simulink model "RM3_Hydraulic_PTO"  (R2019b)
settings: Solver=ode14x  StartTime=0  StopTime=200  FixedStep=0.0025  MaxStep=0.0025  RelTol=1e-3  EnableMultiTasking=on
undefined symbols (not defined in the file or in its folder): body, DiscIntNeverNeededParam, pto
libraries: fl_lib x1519, nesl_utility x807, sh_lib x675, WECSim_Lib x5
(part 16 of 56)

== system RM3_Hydraulic_PTO/PTO-Sim - Crankshaft DA 4 Cylinders Try 4 WORKS - PR valve no ACCUM - No piston control/Cylinder 2 ==
  Crank Radius : Inport
  Spool Radius : Inport  Port=2
  Angle Displacement : Inport  Port=3
  Crank Init Angle : Inport  Port=4
  Crank Torque [Nm] : Product
  Crank Torque [Nm] Sensor : Scope
  Cyl1 Force Sensor : Scope
  Cylinder 1 to PTO Force convert : Subsystem
  Hydraulic cylinder and valves : Subsystem
  Ideal Translational Motion Sensor : fl_lib/Mechanical/Mechanical Sensors/Ideal Translational Motion Sensor  offset=0 m
  Mass : fl_lib/Mechanical/Translational Elements/Mass  mass=1 kg  v_specify=off  v_priority=High  v=0 m/s  v_nominal_specify=off  v_nominal_unit=m/s  v_nominal_value=1  f_specify=off  f_priority=None  f=0 N  f_nominal_specify=off  f_nominal_unit=N  f_nominal_value=1
  PTO Force Cyl 1 Sensor : Scope
  Slider-Crank : fl_lib/Mechanical/Mechanisms/Slider-Crank  crank=11/2 in  rod=12 in  inertia=0.01 kg*m^2  k=1e6 N/m  b=0.0001 N/(m/s)  theta_specify=on  theta_priority=High  theta=0 rad  theta_nominal_specify=off  theta_nominal_unit=rad  theta_nominal_value=1  w_specify=off  w_priority=Low  w=0 rad/s  w_nominal_specify=off  w_nominal_unit=rad/s  w_nominal_value=1
      settings: SourceProductName=Simscape  SourceProductBaseCode=SS  InternalSimscapePortConfiguration="{\"Bottom\":[],\"Left\":[{\"id\":\"C\",\"label\":\"C\",\"type\":\"foundation.mechanical.rotational.rotational\"}],\"Right\":[{\"id\":\"S\",\"label\":\"S\",\"type\":\"foundation.mechanical.translational.translational\"}],\"Top\":[]}"
  Theta sensor : Scope
  sin(theta) sensor : Scope
  Angular Vel Source : PMIOPort  Side=Left
  Flow Out : PMIOPort  Port=2  Side=Left
  Flow In : PMIOPort  Port=3  Side=Left
  PTO Force : Outport
  wires:
  Crank Torque [Nm]/1 -> Crank Torque [Nm] Sensor/1
  Hydraulic cylinder and valves/1(Force Out) -> Cylinder 1 to PTO Force convert/5(Cylinder Force), Cyl1 Force Sensor/1
  Crank Radius/1 -> Cylinder 1 to PTO Force convert/1(Crank radius), Crank Torque [Nm]/1
  Cylinder 1 to PTO Force convert/3(PTO Force Cyl) -> PTO Force/1, Crank Torque [Nm]/2, PTO Force Cyl 1 Sensor/1
  Cylinder 1 to PTO Force convert/2(sing(theta)) -> sin(theta) sensor/1
  Spool Radius/1 -> Cylinder 1 to PTO Force convert/4(Spool radius)
  Cylinder 1 to PTO Force convert/1(Theta) -> Theta sensor/1
  Crank Init Angle/1 -> Cylinder 1 to PTO Force convert/2(Crank initial angle)
  Angle Displacement/1 -> Cylinder 1 to PTO Force convert/3(Angle disp)
  connections:
  Hydraulic cylinder and valves/LConn1 -- Ideal Translational Motion Sensor/RConn2
  Mass/LConn1 -- Ideal Translational Motion Sensor/RConn1
  Slider-Crank/RConn1 -- Ideal Translational Motion Sensor/LConn1
  Slider-Crank/LConn1 -- Angular Vel Source/RConn1
  Flow In/RConn1 -- Hydraulic cylinder and valves/LConn3
  Hydraulic cylinder and valves/LConn2 -- Flow Out/RConn1

== system RM3_Hydraulic_PTO/PTO-Sim - Crankshaft DA 4 Cylinders Try 4 WORKS - PR valve no ACCUM - No piston control/Cylinder 3 ==
  Crank Radius : Inport
  Spool Radius : Inport  Port=2
  Angle Displacement : Inport  Port=3
  Crank Init Angle : Inport  Port=4
  Crank Torque [Nm] : Product
  Crank Torque [Nm] Sensor : Scope
  Cyl1 Force Sensor : Scope
  Cylinder 1 to PTO Force convert : Subsystem
  Hydraulic cylinder and valves : Subsystem
  Ideal Translational Motion Sensor : fl_lib/Mechanical/Mechanical Sensors/Ideal Translational Motion Sensor  offset=0 m
  Mass : fl_lib/Mechanical/Translational Elements/Mass  mass=1 kg  v_specify=off  v_priority=High  v=0 m/s  v_nominal_specify=off  v_nominal_unit=m/s  v_nominal_value=1  f_specify=off  f_priority=None  f=0 N  f_nominal_specify=off  f_nominal_unit=N  f_nominal_value=1
  PTO Force Cyl 1 Sensor : Scope
  Slider-Crank : fl_lib/Mechanical/Mechanisms/Slider-Crank  crank=11/2 in  rod=12 in  inertia=0.01 kg*m^2  k=1e6 N/m  b=0.0001 N/(m/s)  theta_specify=on  theta_priority=High  theta=3*pi/2 rad  theta_nominal_specify=off  theta_nominal_unit=rad  theta_nominal_value=1  w_specify=off  w_priority=Low  w=0 rad/s  w_nominal_specify=off  w_nominal_unit=rad/s  w_nominal_value=1
      settings: SourceProductName=Simscape  SourceProductBaseCode=SS  InternalSimscapePortConfiguration="{\"Bottom\":[],\"Left\":[{\"id\":\"C\",\"label\":\"C\",\"type\":\"foundation.mechanical.rotational.rotational\"}],\"Right\":[{\"id\":\"S\",\"label\":\"S\",\"type\":\"foundation.mechanical.translational.translational\"}],\"Top\":[]}"
  Theta sensor : Scope
  sin(theta) sensor : Scope
  Angular Vel Source : PMIOPort  Side=Left
  Flow Out : PMIOPort  Port=2  Side=Left
  Flow In : PMIOPort  Port=3  Side=Left
  PTO Force : Outport
  wires:
  Crank Torque [Nm]/1 -> Crank Torque [Nm] Sensor/1
  Hydraulic cylinder and valves/1(Force Out) -> Cylinder 1 to PTO Force convert/5(Cylinder Force), Cyl1 Force Sensor/1
  Crank Radius/1 -> Cylinder 1 to PTO Force convert/1(Crank radius), Crank Torque [Nm]/1
  Cylinder 1 to PTO Force convert/3(PTO Force Cyl) -> PTO Force/1, Crank Torque [Nm]/2, PTO Force Cyl 1 Sensor/1
  Cylinder 1 to PTO Force convert/2(sing(theta)) -> sin(theta) sensor/1
  Spool Radius/1 -> Cylinder 1 to PTO Force convert/4(Spool radius)
  Cylinder 1 to PTO Force convert/1(Theta) -> Theta sensor/1
  Crank Init Angle/1 -> Cylinder 1 to PTO Force convert/2(Crank initial angle)
  Angle Displacement/1 -> Cylinder 1 to PTO Force convert/3(Angle disp)
  connections:
  Hydraulic cylinder and valves/LConn1 -- Ideal Translational Motion Sensor/RConn2
  Mass/LConn1 -- Ideal Translational Motion Sensor/RConn1
  Slider-Crank/RConn1 -- Ideal Translational Motion Sensor/LConn1
  Slider-Crank/LConn1 -- Angular Vel Source/RConn1
  Flow In/RConn1 -- Hydraulic cylinder and valves/LConn3
  Hydraulic cylinder and valves/LConn2 -- Flow Out/RConn1

== system RM3_Hydraulic_PTO/PTO-Sim - Crankshaft DA 4 Cylinders Try 4 WORKS - PR valve no ACCUM - No piston control/Cylinder 4 ==
  Crank Radius : Inport
  Spool Radius : Inport  Port=2
  Angle Displacement : Inport  Port=3
  Crank Init Angle : Inport  Port=4
  Crank Torque [Nm] : Product
  Crank Torque [Nm] Sensor : Scope
  Cyl1 Force Sensor : Scope
  Cylinder 1 to PTO Force convert : Subsystem
  Hydraulic cylinder and valves : Subsystem
  Ideal Translational Motion Sensor : fl_lib/Mechanical/Mechanical Sensors/Ideal Translational Motion Sensor  offset=0 m
  Mass : fl_lib/Mechanical/Translational Elements/Mass  mass=1 kg  v_specify=off  v_priority=High  v=0 m/s  v_nominal_specify=off  v_nominal_unit=m/s  v_nominal_value=1  f_specify=off  f_priority=None  f=0 N  f_nominal_specify=off  f_nominal_unit=N  f_nominal_value=1
  PTO Force Cyl 1 Sensor : Scope
  Slider-Crank : fl_lib/Mechanical/Mechanisms/Slider-Crank  crank=11/2 in  rod=12 in  inertia=0.01 kg*m^2  k=1e6 N/m  b=0.0001 N/(m/s)  theta_specify=on  theta_priority=High  theta=pi rad  theta_nominal_specify=off  theta_nominal_unit=rad  theta_nominal_value=1  w_specify=off  w_priority=Low  w=0 rad/s  w_nominal_specify=off  w_nominal_unit=rad/s  w_nominal_value=1
      settings: SourceProductName=Simscape  SourceProductBaseCode=SS  InternalSimscapePortConfiguration="{\"Bottom\":[],\"Left\":[{\"id\":\"C\",\"label\":\"C\",\"type\":\"foundation.mechanical.rotational.rotational\"}],\"Right\":[{\"id\":\"S\",\"label\":\"S\",\"type\":\"foundation.mechanical.translational.translational\"}],\"Top\":[]}"
  Theta sensor : Scope
  sin(theta) sensor : Scope
  Angular Vel Source : PMIOPort  Side=Left
  Flow Out : PMIOPort  Port=2  Side=Left
  Flow In : PMIOPort  Port=3  Side=Left
  PTO Force : Outport
  wires:
  Crank Torque [Nm]/1 -> Crank Torque [Nm] Sensor/1
  Hydraulic cylinder and valves/1(Force Out) -> Cylinder 1 to PTO Force convert/5(Cylinder Force), Cyl1 Force Sensor/1
  Crank Radius/1 -> Cylinder 1 to PTO Force convert/1(Crank radius), Crank Torque [Nm]/1
  Cylinder 1 to PTO Force convert/3(PTO Force Cyl) -> PTO Force/1, Crank Torque [Nm]/2, PTO Force Cyl 1 Sensor/1
  Cylinder 1 to PTO Force convert/2(sing(theta)) -> sin(theta) sensor/1
  Spool Radius/1 -> Cylinder 1 to PTO Force convert/4(Spool radius)
  Cylinder 1 to PTO Force convert/1(Theta) -> Theta sensor/1
  Crank Init Angle/1 -> Cylinder 1 to PTO Force convert/2(Crank initial angle)
  Angle Displacement/1 -> Cylinder 1 to PTO Force convert/3(Angle disp)
  connections:
  Hydraulic cylinder and valves/LConn1 -- Ideal Translational Motion Sensor/RConn2
  Mass/LConn1 -- Ideal Translational Motion Sensor/RConn1
  Slider-Crank/RConn1 -- Ideal Translational Motion Sensor/LConn1
  Slider-Crank/LConn1 -- Angular Vel Source/RConn1
  Flow In/RConn1 -- Hydraulic cylinder and valves/LConn3
  Hydraulic cylinder and valves/LConn2 -- Flow Out/RConn1

== system RM3_Hydraulic_PTO/PTO-Sim - Crankshaft DA 4 Cylinders Try 4 WORKS - PR valve no ACCUM - No piston control/RO Membrane ==
  " Flow Rate Feed Sensor" : fl_lib/Hydraulic/Hydraulic Sensors/Hydraulic Flow Rate Sensor
      settings: SourceProductName=Simscape
  Brine : fl_lib/Hydraulic/Hydraulic Elements/Hydraulic Reference
      settings: SourceProductName=Simscape
  Brine1 : fl_lib/Hydraulic/Hydraulic Elements/Hydraulic Reference
      settings: SourceProductName=Simscape
  Flow Rate Brine Sensor : fl_lib/Hydraulic/Hydraulic Sensors/Hydraulic Flow Rate Sensor
      settings: SourceProductName=Simscape
  Flow Rate Permeate Sensor : fl_lib/Hydraulic/Hydraulic Sensors/Hydraulic Flow Rate Sensor
      settings: SourceProductName=Simscape
  Flow Restrictor : fl_lib/Hydraulic/Hydraulic Elements/Linear Hydraulic Resistance  resistance=(0.20) * ( 1/((3.812*10^-12)*(7.4 ) ) ) Pa/(m^3/s)  q_specify=off  q_priority=None  q=0.001 m^3/s  q_nominal_specify=off  q_nominal_unit=m^3/s  q_nominal_value=1  p_specify=off  p_priority=None  p=0 Pa  p_nominal_specify=off  p_nominal_unit=Pa  p_nominal_value=1
      settings: SourceProductName=Simscape  SourceProductBaseCode=SS  InternalSimscapePortConfiguration="{\"Bottom\":[],\"Left\":[{\"id\":\"A\",\"label\":\"A\",\"type\":\"foundation.hydraulic.hydraulic\"}],\"Right\":[{\"id\":\"B\",\"label\":\"B\",\"type\":\"foundation.hydraulic.hydraulic\"}],\"Top\":[]}"
  Osmotic Pressure 1 : sh_lib/Valves/Pressure Control Valves/Pressure Relief Valve  valve_area_spec=1  p_diff_TLU=[30.15e5 : 15e3 : 31.35e5] Pa  area_TLU=[1 : 1 : 9] .* 1e-5 m^2  area_max=10*pi*(0.75/2)^2 in^2  pres_set=30 bar  reg_range=2 bar  C_d=0.7  A_leak=1e-12 m^2  lam_spec=1  B_lam=0.999  Re_cr=12  dynamic=0  tau=0.1 s  area_init=1e-12 m^2
      settings: SourceProductName=Simscape Fluids  SourceProductBaseCode=SH  InternalSimscapePortConfiguration="{\"Bottom\":[],\"Left\":[{\"id\":\"A\",\"label\":\"A\",\"type\":\"foundation.hydraulic.hydraulic\"}],\"Right\":[{\"id\":\"B\",\"label\":\"B\",\"type\":\"foundation.hydraulic.hydraulic\"}],\"Top\":[]}"
  P Brine Exit : Scope
  PS Subtract : fl_lib/Physical Signals/Functions/PS Subtract
      settings: SourceProductName=Simscape
  PS-Simulink Converter7 : nesl_utility/PS-Simulink Converter  PhysicalDomain=network_engine_domain  SubClassName=ps_output  LeftPortType=input  RightPortType=output  PseudoPeriodic=off  Frequencies=[]  Unit=inherit  AffineConversion=off
  Permeate : fl_lib/Hydraulic/Hydraulic Elements/Hydraulic Reference
      settings: SourceProductName=Simscape
  Pressure Drop Brine : fl_lib/Hydraulic/Hydraulic Sensors/Hydraulic Pressure Sensor
      settings: SourceProductName=Simscape
  Pressure Drop Permeate : fl_lib/Hydraulic/Hydraulic Sensors/Hydraulic Pressure Sensor
      settings: SourceProductName=Simscape
  Pressure Perm Before : fl_lib/Hydraulic/Hydraulic Sensors/Hydraulic Pressure Sensor
      settings: SourceProductName=Simscape
  Pressure Sensor Brine1 : fl_lib/Hydraulic/Hydraulic Sensors/Hydraulic Pressure Sensor
      settings: SourceProductName=Simscape
  Pressure Sensor Feed : fl_lib/Hydraulic/Hydraulic Sensors/Hydraulic Pressure Sensor
      settings: SourceProductName=Simscape
  RO Membrane1 : fl_lib/Hydraulic/Hydraulic Elements/Linear Hydraulic Resistance  resistance=1/((3.812*10^-12)*(7.4 ) ) Pa/(m^3/s)  q_specify=off  q_priority=None  q=0.001 m^3/s  q_nominal_specify=off  q_nominal_unit=m^3/s  q_nominal_value=1  p_specify=off  p_priority=None  p=0 Pa  p_nominal_specify=off  p_nominal_unit=Pa  p_nominal_value=1
      settings: SourceProductName=Simscape  SourceProductBaseCode=SS  InternalSimscapePortConfiguration="{\"Bottom\":[],\"Left\":[{\"id\":\"A\",\"label\":\"A\",\"type\":\"foundation.hydraulic.hydraulic\"}],\"Right\":[{\"id\":\"B\",\"label\":\"B\",\"type\":\"foundation.hydraulic.hydraulic\"}],\"Top\":[]}"
  Ref1 : fl_lib/Hydraulic/Hydraulic Elements/Hydraulic Reference
      settings: SourceProductName=Simscape
  Ref2 : fl_lib/Hydraulic/Hydraulic Elements/Hydraulic Reference
      settings: SourceProductName=Simscape
  Pressure Perm before RO : PMIOPort  Side=Right
  Pressure Drop Perm : PMIOPort  Port=2  Side=Right
  Flow rate feed : PMIOPort  Port=3  Side=Right
  Flow rate permeate : PMIOPort  Port=4  Side=Right
  Pressure Feed : PMIOPort  Port=5  Side=Right
  Flow in : PMIOPort  Port=6  Side=Left
  Mass flow rate feed : PMIOPort  Port=7  Side=Right
  Mass Flow rate perm : PMIOPort  Port=8  Side=Right
  Flow rate brine : PMIOPort  Port=9  Side=Right
  Mass flow rate brine : PMIOPort  Port=10  Side=Right
  wires:
  PS-Simulink Converter7/1 -> P Brine Exit/1
  connections:
  RO Membrane1/RConn1 -- Pressure Drop Permeate/RConn1 -- Flow Rate Permeate Sensor/LConn1
  " Flow Rate Feed Sensor"/RConn2 -- Pressure Sensor Brine1/LConn1 -- Pressure Drop Brine/LConn1 -- Flow Restrictor/LConn1 -- Osmotic Pressure 1/LConn1
  Pressure Drop Permeate/LConn1 -- RO Membrane1/LConn1 -- Osmotic Pressure 1/RConn1 -- Pressure Perm Before/LConn1
  Pressure Perm Before/RConn1 -- Ref2/LConn1
  Flow Rate Brine Sensor/LConn1 -- Pressure Drop Brine/RConn1 -- Flow Restrictor/RConn1
  " Flow Rate Feed Sensor"/LConn1 -- Pressure Sensor Feed/LConn1 -- Flow in/RConn1
  Flow Rate Permeate Sensor/RConn2 -- Permeate/LConn1
  Pressure Sensor Brine1/RConn1 -- Brine1/LConn1
  " Flow Rate Feed Sensor"/RConn1 -- Flow rate feed/RConn1
  PS Subtract/RConn1 -- PS-Simulink Converter7/LConn1
  Pressure Sensor Feed/RConn2 -- Pressure Feed/RConn1
  Flow Rate Brine Sensor/RConn2 -- Brine/LConn1
  Pressure Sensor Feed/RConn1 -- Ref1/LConn1
  Flow Rate Permeate Sensor/RConn1 -- Flow rate permeate/RConn1
  Pressure Perm before RO/RConn1 -- Pressure Perm Before/RConn2
  Pressure Drop Brine/RConn2 -- PS Subtract/LConn2
  Pressure Sensor Brine1/RConn2 -- PS Subtract/LConn1
  Pressure Drop Permeate/RConn2 -- Pressure Drop Perm/RConn1
  " Flow Rate Feed Sensor"/RConn3 -- Mass flow rate feed/RConn1
  Flow Rate Permeate Sensor/RConn3 -- Mass Flow rate perm/RConn1
  Flow Rate Brine Sensor/RConn1 -- Flow rate brine/RConn1
  Flow Rate Brine Sensor/RConn3 -- Mass flow rate brine/RConn1

== system RM3_Hydraulic_PTO/PTO-Sim - Crankshaft DA 4 Cylinders Try 5 - Cylinder shutoff control - 1/Cylinder 1 ==
  Crank Radius : Inport
  Spool Radius : Inport  Port=2
  Angle Displacement : Inport  Port=3
  Crank Init Angle : Inport  Port=4
  Crank Torque [Nm] : Product
  Crank Torque [Nm] Sensor : Scope
  Cyl1 Force Sensor : Scope
  Cylinder 1 to PTO Force convert : Subsystem
  Hydraulic cylinder and valves : Subsystem
  Ideal Translational Motion Sensor : fl_lib/Mechanical/Mechanical Sensors/Ideal Translational Motion Sensor  offset=0 m
  Mass : fl_lib/Mechanical/Translational Elements/Mass  mass=1 kg  v_specify=off  v_priority=High  v=0 m/s  v_nominal_specify=off  v_nominal_unit=m/s  v_nominal_value=1  f_specify=off  f_priority=None  f=0 N  f_nominal_specify=off  f_nominal_unit=N  f_nominal_value=1
  PTO Force Cyl 1 Sensor : Scope
  Slider-Crank : fl_lib/Mechanical/Mechanisms/Slider-Crank  crank=11/2 in  rod=12 in  inertia=0.01 kg*m^2  k=1e6 N/m  b=0.0001 N/(m/s)  theta_specify=on  theta_priority=High  theta=pi / 2 rad  theta_nominal_specify=off  theta_nominal_unit=rad  theta_nominal_value=1  w_specify=off  w_priority=Low  w=0 rad/s  w_nominal_specify=off  w_nominal_unit=rad/s  w_nominal_value=1
      settings: SourceProductName=Simscape  SourceProductBaseCode=SS  InternalSimscapePortConfiguration="{\"Bottom\":[],\"Left\":[{\"id\":\"C\",\"label\":\"C\",\"type\":\"foundation.mechanical.rotational.rotational\"}],\"Right\":[{\"id\":\"S\",\"label\":\"S\",\"type\":\"foundation.mechanical.translational.translational\"}],\"Top\":[]}"
  Theta sensor : Scope
  sin(theta) sensor : Scope
  Angular Vel Source : PMIOPort  Side=Left
  Flow Out : PMIOPort  Port=2  Side=Left
  Flow In : PMIOPort  Port=3  Side=Left
  PTO Force : Outport
  wires:
  Crank Torque [Nm]/1 -> Crank Torque [Nm] Sensor/1
  Hydraulic cylinder and valves/1(Force Out) -> Cylinder 1 to PTO Force convert/5(Cylinder Force), Cyl1 Force Sensor/1
  Crank Radius/1 -> Cylinder 1 to PTO Force convert/1(Crank radius), Crank Torque [Nm]/1
  Cylinder 1 to PTO Force convert/3(PTO Force Cyl) -> PTO Force/1, Crank Torque [Nm]/2, PTO Force Cyl 1 Sensor/1
  Cylinder 1 to PTO Force convert/2(sing(theta)) -> sin(theta) sensor/1
  Spool Radius/1 -> Cylinder 1 to PTO Force convert/4(Spool radius)
  Cylinder 1 to PTO Force convert/1(Theta) -> Theta sensor/1
  Crank Init Angle/1 -> Cylinder 1 to PTO Force convert/2(Crank initial angle)
  Angle Displacement/1 -> Cylinder 1 to PTO Force convert/3(Angle disp)
  connections:
  Hydraulic cylinder and valves/LConn1 -- Ideal Translational Motion Sensor/RConn2
  Mass/LConn1 -- Ideal Translational Motion Sensor/RConn1
  Slider-Crank/RConn1 -- Ideal Translational Motion Sensor/LConn1
  Slider-Crank/LConn1 -- Angular Vel Source/RConn1
  Flow In/RConn1 -- Hydraulic cylinder and valves/LConn3
  Hydraulic cylinder and valves/LConn2 -- Flow Out/RConn1

== system RM3_Hydraulic_PTO/PTO-Sim - Crankshaft DA 4 Cylinders Try 5 - Cylinder shutoff control - 1/Cylinder 2 ==
  Crank Radius : Inport
  Spool Radius : Inport  Port=2
  Angle Displacement : Inport  Port=3
  Crank Init Angle : Inport  Port=4
  Crank Torque [Nm] : Product
  Crank Torque [Nm] Sensor : Scope
  Cyl1 Force Sensor : Scope
  Cylinder 1 to PTO Force convert : Subsystem
  Hydraulic cylinder and valves : Subsystem
  Ideal Translational Motion Sensor : fl_lib/Mechanical/Mechanical Sensors/Ideal Translational Motion Sensor  offset=0 m
  Mass : fl_lib/Mechanical/Translational Elements/Mass  mass=1 kg  v_specify=off  v_priority=High  v=0 m/s  v_nominal_specify=off  v_nominal_unit=m/s  v_nominal_value=1  f_specify=off  f_priority=None  f=0 N  f_nominal_specify=off  f_nominal_unit=N  f_nominal_value=1
  PTO Force Cyl 1 Sensor : Scope
  Slider-Crank : fl_lib/Mechanical/Mechanisms/Slider-Crank  crank=11/2 in  rod=12 in  inertia=0.01 kg*m^2  k=1e6 N/m  b=0.0001 N/(m/s)  theta_specify=on  theta_priority=High  theta=0 rad  theta_nominal_specify=off  theta_nominal_unit=rad  theta_nominal_value=1  w_specify=off  w_priority=Low  w=0 rad/s  w_nominal_specify=off  w_nominal_unit=rad/s  w_nominal_value=1
      settings: SourceProductName=Simscape  SourceProductBaseCode=SS  InternalSimscapePortConfiguration="{\"Bottom\":[],\"Left\":[{\"id\":\"C\",\"label\":\"C\",\"type\":\"foundation.mechanical.rotational.rotational\"}],\"Right\":[{\"id\":\"S\",\"label\":\"S\",\"type\":\"foundation.mechanical.translational.translational\"}],\"Top\":[]}"
  Theta sensor : Scope
  sin(theta) sensor : Scope
  Angular Vel Source : PMIOPort  Side=Left
  Flow Out : PMIOPort  Port=2  Side=Left
  Flow In : PMIOPort  Port=3  Side=Left
  PTO Force : Outport
  wires:
  Crank Torque [Nm]/1 -> Crank Torque [Nm] Sensor/1
  Hydraulic cylinder and valves/1(Force Out) -> Cylinder 1 to PTO Force convert/5(Cylinder Force), Cyl1 Force Sensor/1
  Crank Radius/1 -> Cylinder 1 to PTO Force convert/1(Crank radius), Crank Torque [Nm]/1
  Cylinder 1 to PTO Force convert/3(PTO Force Cyl) -> PTO Force/1, Crank Torque [Nm]/2, PTO Force Cyl 1 Sensor/1
  Cylinder 1 to PTO Force convert/2(sing(theta)) -> sin(theta) sensor/1
  Spool Radius/1 -> Cylinder 1 to PTO Force convert/4(Spool radius)
  Cylinder 1 to PTO Force convert/1(Theta) -> Theta sensor/1
  Crank Init Angle/1 -> Cylinder 1 to PTO Force convert/2(Crank initial angle)
  Angle Displacement/1 -> Cylinder 1 to PTO Force convert/3(Angle disp)
  connections:
  Hydraulic cylinder and valves/LConn1 -- Ideal Translational Motion Sensor/RConn2
  Mass/LConn1 -- Ideal Translational Motion Sensor/RConn1
  Slider-Crank/RConn1 -- Ideal Translational Motion Sensor/LConn1
  Slider-Crank/LConn1 -- Angular Vel Source/RConn1
  Flow In/RConn1 -- Hydraulic cylinder and valves/LConn3
  Hydraulic cylinder and valves/LConn2 -- Flow Out/RConn1

== system RM3_Hydraulic_PTO/PTO-Sim - Crankshaft DA 4 Cylinders Try 5 - Cylinder shutoff control - 1/Cylinder 3 ==
  Crank Radius : Inport
  Spool Radius : Inport  Port=2
  Angle Displacement : Inport  Port=3
  Crank Init Angle : Inport  Port=4
  Crank Torque [Nm] : Product
  Crank Torque [Nm] Sensor : Scope
  Cyl1 Force Sensor : Scope
  Cylinder 1 to PTO Force convert : Subsystem
  Hydraulic cylinder and valves : Subsystem
  Ideal Translational Motion Sensor : fl_lib/Mechanical/Mechanical Sensors/Ideal Translational Motion Sensor  offset=0 m
  Mass : fl_lib/Mechanical/Translational Elements/Mass  mass=1 kg  v_specify=off  v_priority=High  v=0 m/s  v_nominal_specify=off  v_nominal_unit=m/s  v_nominal_value=1  f_specify=off  f_priority=None  f=0 N  f_nominal_specify=off  f_nominal_unit=N  f_nominal_value=1
  PTO Force Cyl 1 Sensor : Scope
  Slider-Crank : fl_lib/Mechanical/Mechanisms/Slider-Crank  crank=11/2 in  rod=12 in  inertia=0.01 kg*m^2  k=1e6 N/m  b=0.0001 N/(m/s)  theta_specify=on  theta_priority=High  theta=3*pi/2 rad  theta_nominal_specify=off  theta_nominal_unit=rad  theta_nominal_value=1  w_specify=off  w_priority=Low  w=0 rad/s  w_nominal_specify=off  w_nominal_unit=rad/s  w_nominal_value=1
      settings: SourceProductName=Simscape  SourceProductBaseCode=SS  InternalSimscapePortConfiguration="{\"Bottom\":[],\"Left\":[{\"id\":\"C\",\"label\":\"C\",\"type\":\"foundation.mechanical.rotational.rotational\"}],\"Right\":[{\"id\":\"S\",\"label\":\"S\",\"type\":\"foundation.mechanical.translational.translational\"}],\"Top\":[]}"
  Theta sensor : Scope
  sin(theta) sensor : Scope
  Angular Vel Source : PMIOPort  Side=Left
  Flow Out : PMIOPort  Port=2  Side=Left
  Flow In : PMIOPort  Port=3  Side=Left
  PTO Force : Outport
  wires:
  Crank Torque [Nm]/1 -> Crank Torque [Nm] Sensor/1
  Hydraulic cylinder and valves/1(Force Out) -> Cylinder 1 to PTO Force convert/5(Cylinder Force), Cyl1 Force Sensor/1
  Crank Radius/1 -> Cylinder 1 to PTO Force convert/1(Crank radius), Crank Torque [Nm]/1
  Cylinder 1 to PTO Force convert/3(PTO Force Cyl) -> PTO Force/1, Crank Torque [Nm]/2, PTO Force Cyl 1 Sensor/1
  Cylinder 1 to PTO Force convert/2(sing(theta)) -> sin(theta) sensor/1
  Spool Radius/1 -> Cylinder 1 to PTO Force convert/4(Spool radius)
  Cylinder 1 to PTO Force convert/1(Theta) -> Theta sensor/1
  Crank Init Angle/1 -> Cylinder 1 to PTO Force convert/2(Crank initial angle)
  Angle Displacement/1 -> Cylinder 1 to PTO Force convert/3(Angle disp)
  connections:
  Hydraulic cylinder and valves/LConn1 -- Ideal Translational Motion Sensor/RConn2
  Mass/LConn1 -- Ideal Translational Motion Sensor/RConn1
  Slider-Crank/RConn1 -- Ideal Translational Motion Sensor/LConn1
  Slider-Crank/LConn1 -- Angular Vel Source/RConn1
  Flow In/RConn1 -- Hydraulic cylinder and valves/LConn3
  Hydraulic cylinder and valves/LConn2 -- Flow Out/RConn1

== system RM3_Hydraulic_PTO/PTO-Sim - Crankshaft DA 4 Cylinders Try 5 - Cylinder shutoff control - 1/Cylinder 4 ==
  Crank Radius : Inport
  Spool Radius : Inport  Port=2
  Angle Displacement : Inport  Port=3
  Crank Init Angle : Inport  Port=4
  Crank Torque [Nm] : Product
  Crank Torque [Nm] Sensor : Scope
  Cyl1 Force Sensor : Scope
  Cylinder 1 to PTO Force convert : Subsystem
  Hydraulic cylinder and valves : Subsystem
  Ideal Translational Motion Sensor : fl_lib/Mechanical/Mechanical Sensors/Ideal Translational Motion Sensor  offset=0 m
  Mass : fl_lib/Mechanical/Translational Elements/Mass  mass=1 kg  v_specify=off  v_priority=High  v=0 m/s  v_nominal_specify=off  v_nominal_unit=m/s  v_nominal_value=1  f_specify=off  f_priority=None  f=0 N  f_nominal_specify=off  f_nominal_unit=N  f_nominal_value=1
  PTO Force Cyl 1 Sensor : Scope
  Slider-Crank : fl_lib/Mechanical/Mechanisms/Slider-Crank  crank=11/2 in  rod=12 in  inertia=0.01 kg*m^2  k=1e6 N/m  b=0.0001 N/(m/s)  theta_specify=on  theta_priority=High  theta=pi rad  theta_nominal_specify=off  theta_nominal_unit=rad  theta_nominal_value=1  w_specify=off  w_priority=Low  w=0 rad/s  w_nominal_specify=off  w_nominal_unit=rad/s  w_nominal_value=1
      settings: SourceProductName=Simscape  SourceProductBaseCode=SS  InternalSimscapePortConfiguration="{\"Bottom\":[],\"Left\":[{\"id\":\"C\",\"label\":\"C\",\"type\":\"foundation.mechanical.rotational.rotational\"}],\"Right\":[{\"id\":\"S\",\"label\":\"S\",\"type\":\"foundation.mechanical.translational.translational\"}],\"Top\":[]}"
  Theta sensor : Scope
  sin(theta) sensor : Scope
  Angular Vel Source : PMIOPort  Side=Left
  Flow Out : PMIOPort  Port=2  Side=Left
  Flow In : PMIOPort  Port=3  Side=Left
  PTO Force : Outport
  wires:
  Crank Torque [Nm]/1 -> Crank Torque [Nm] Sensor/1
  Hydraulic cylinder and valves/1(Force Out) -> Cylinder 1 to PTO Force convert/5(Cylinder Force), Cyl1 Force Sensor/1
  Crank Radius/1 -> Cylinder 1 to PTO Force convert/1(Crank radius), Crank Torque [Nm]/1
  Cylinder 1 to PTO Force convert/3(PTO Force Cyl) -> PTO Force/1, Crank Torque [Nm]/2, PTO Force Cyl 1 Sensor/1
  Cylinder 1 to PTO Force convert/2(sing(theta)) -> sin(theta) sensor/1
  Spool Radius/1 -> Cylinder 1 to PTO Force convert/4(Spool radius)
  Cylinder 1 to PTO Force convert/1(Theta) -> Theta sensor/1
  Crank Init Angle/1 -> Cylinder 1 to PTO Force convert/2(Crank initial angle)
  Angle Displacement/1 -> Cylinder 1 to PTO Force convert/3(Angle disp)
  connections:
  Hydraulic cylinder and valves/LConn1 -- Ideal Translational Motion Sensor/RConn2
  Mass/LConn1 -- Ideal Translational Motion Sensor/RConn1
  Slider-Crank/RConn1 -- Ideal Translational Motion Sensor/LConn1
  Slider-Crank/LConn1 -- Angular Vel Source/RConn1
  Flow In/RConn1 -- Hydraulic cylinder and valves/LConn3
  Hydraulic cylinder and valves/LConn2 -- Flow Out/RConn1

== system RM3_Hydraulic_PTO/PTO-Sim - Crankshaft DA 4 Cylinders Try 5 - Cylinder shutoff control - 1/RO Membrane ==
  " Flow Rate Feed Sensor" : fl_lib/Hydraulic/Hydraulic Sensors/Hydraulic Flow Rate Sensor
      settings: SourceProductName=Simscape
  Brine : fl_lib/Hydraulic/Hydraulic Elements/Hydraulic Reference
      settings: SourceProductName=Simscape
  Brine1 : fl_lib/Hydraulic/Hydraulic Elements/Hydraulic Reference
      settings: SourceProductName=Simscape
  Flow Rate Brine Sensor : fl_lib/Hydraulic/Hydraulic Sensors/Hydraulic Flow Rate Sensor
      settings: SourceProductName=Simscape
  Flow Rate Permeate Sensor : fl_lib/Hydraulic/Hydraulic Sensors/Hydraulic Flow Rate Sensor
      settings: SourceProductName=Simscape
  Flow Restrictor : fl_lib/Hydraulic/Hydraulic Elements/Linear Hydraulic Resistance  resistance=(0.30) * ( 1/((3.812*10^-12)*(7.4 ) ) ) Pa/(m^3/s)  q_specify=off  q_priority=None  q=0.001 m^3/s  q_nominal_specify=off  q_nominal_unit=m^3/s  q_nominal_value=1  p_specify=off  p_priority=None  p=0 Pa  p_nominal_specify=off  p_nominal_unit=Pa  p_nominal_value=1
      settings: SourceProductName=Simscape  SourceProductBaseCode=SS  InternalSimscapePortConfiguration="{\"Bottom\":[],\"Left\":[{\"id\":\"A\",\"label\":\"A\",\"type\":\"foundation.hydraulic.hydraulic\"}],\"Right\":[{\"id\":\"B\",\"label\":\"B\",\"type\":\"foundation.hydraulic.hydraulic\"}],\"Top\":[]}"
  Osmotic Pressure 1 : sh_lib/Valves/Pressure Control Valves/Pressure Relief Valve  valve_area_spec=1  p_diff_TLU=[30.15e5 : 15e3 : 31.35e5] Pa  area_TLU=[1 : 1 : 9] .* 1e-5 m^2  area_max=10*pi*(0.75/2)^2 in^2  pres_set=30 bar  reg_range=2 bar  C_d=0.7  A_leak=1e-12 m^2  lam_spec=1  B_lam=0.999  Re_cr=12  dynamic=0  tau=0.1 s  area_init=1e-12 m^2
      settings: SourceProductName=Simscape Fluids  SourceProductBaseCode=SH  InternalSimscapePortConfiguration="{\"Bottom\":[],\"Left\":[{\"id\":\"A\",\"label\":\"A\",\"type\":\"foundation.hydraulic.hydraulic\"}],\"Right\":[{\"id\":\"B\",\"label\":\"B\",\"type\":\"foundation.hydraulic.hydraulic\"}],\"Top\":[]}"
  P Brine Exit : Scope
  PS Subtract : fl_lib/Physical Signals/Functions/PS Subtract
      settings: SourceProductName=Simscape
  PS-Simulink Converter7 : nesl_utility/PS-Simulink Converter  PhysicalDomain=network_engine_domain  SubClassName=ps_output  LeftPortType=input  RightPortType=output  PseudoPeriodic=off  Frequencies=[]  Unit=inherit  AffineConversion=off
  Permeate : fl_lib/Hydraulic/Hydraulic Elements/Hydraulic Reference
      settings: SourceProductName=Simscape
  Pressure Drop Brine : fl_lib/Hydraulic/Hydraulic Sensors/Hydraulic Pressure Sensor
      settings: SourceProductName=Simscape
  Pressure Drop Permeate : fl_lib/Hydraulic/Hydraulic Sensors/Hydraulic Pressure Sensor
      settings: SourceProductName=Simscape
  Pressure Perm Before : fl_lib/Hydraulic/Hydraulic Sensors/Hydraulic Pressure Sensor
      settings: SourceProductName=Simscape
  Pressure Sensor Brine1 : fl_lib/Hydraulic/Hydraulic Sensors/Hydraulic Pressure Sensor
      settings: SourceProductName=Simscape
  Pressure Sensor Feed : fl_lib/Hydraulic/Hydraulic Sensors/Hydraulic Pressure Sensor
      settings: SourceProductName=Simscape
  RO Membrane1 : fl_lib/Hydraulic/Hydraulic Elements/Linear Hydraulic Resistance  resistance=1/((3.812*10^-12)*(7.4 ) ) Pa/(m^3/s)  q_specify=off  q_priority=None  q=0.001 m^3/s  q_nominal_specify=off  q_nominal_unit=m^3/s  q_nominal_value=1  p_specify=off  p_priority=None  p=0 Pa  p_nominal_specify=off  p_nominal_unit=Pa  p_nominal_value=1
      settings: SourceProductName=Simscape  SourceProductBaseCode=SS  InternalSimscapePortConfiguration="{\"Bottom\":[],\"Left\":[{\"id\":\"A\",\"label\":\"A\",\"type\":\"foundation.hydraulic.hydraulic\"}],\"Right\":[{\"id\":\"B\",\"label\":\"B\",\"type\":\"foundation.hydraulic.hydraulic\"}],\"Top\":[]}"
  Ref1 : fl_lib/Hydraulic/Hydraulic Elements/Hydraulic Reference
      settings: SourceProductName=Simscape
  Ref2 : fl_lib/Hydraulic/Hydraulic Elements/Hydraulic Reference
      settings: SourceProductName=Simscape
  Pressure Perm before RO : PMIOPort  Side=Right
  Pressure Drop Perm : PMIOPort  Port=2  Side=Right
  Flow rate feed : PMIOPort  Port=3  Side=Right
  Flow rate permeate : PMIOPort  Port=4  Side=Right
  Pressure Feed : PMIOPort  Port=5  Side=Right
  Flow in : PMIOPort  Port=6  Side=Left
  Mass flow rate feed : PMIOPort  Port=7  Side=Right
  Mass Flow rate perm : PMIOPort  Port=8  Side=Right
  Flow rate brine : PMIOPort  Port=9  Side=Right
  Mass flow rate brine : PMIOPort  Port=10  Side=Right
  wires:
  PS-Simulink Converter7/1 -> P Brine Exit/1
  connections:
  RO Membrane1/RConn1 -- Pressure Drop Permeate/RConn1 -- Flow Rate Permeate Sensor/LConn1
  " Flow Rate Feed Sensor"/RConn2 -- Pressure Sensor Brine1/LConn1 -- Pressure Drop Brine/LConn1 -- Flow Restrictor/LConn1 -- Osmotic Pressure 1/LConn1
  Pressure Drop Permeate/LConn1 -- RO Membrane1/LConn1 -- Osmotic Pressure 1/RConn1 -- Pressure Perm Before/LConn1
  Pressure Perm Before/RConn1 -- Ref2/LConn1
  Flow Rate Brine Sensor/LConn1 -- Pressure Drop Brine/RConn1 -- Flow Restrictor/RConn1
  " Flow Rate Feed Sensor"/LConn1 -- Pressure Sensor Feed/LConn1 -- Flow in/RConn1
  Flow Rate Permeate Sensor/RConn2 -- Permeate/LConn1
  Pressure Sensor Brine1/RConn1 -- Brine1/LConn1
  " Flow Rate Feed Sensor"/RConn1 -- Flow rate feed/RConn1
  PS Subtract/RConn1 -- PS-Simulink Converter7/LConn1
  Pressure Sensor Feed/RConn2 -- Pressure Feed/RConn1
  Flow Rate Brine Sensor/RConn2 -- Brine/LConn1
  Pressure Sensor Feed/RConn1 -- Ref1/LConn1
  Flow Rate Permeate Sensor/RConn1 -- Flow rate permeate/RConn1
  Pressure Perm before RO/RConn1 -- Pressure Perm Before/RConn2
  Pressure Drop Brine/RConn2 -- PS Subtract/LConn2
  Pressure Sensor Brine1/RConn2 -- PS Subtract/LConn1
  Pressure Drop Permeate/RConn2 -- Pressure Drop Perm/RConn1
  " Flow Rate Feed Sensor"/RConn3 -- Mass flow rate feed/RConn1
  Flow Rate Permeate Sensor/RConn3 -- Mass Flow rate perm/RConn1
  Flow Rate Brine Sensor/RConn1 -- Flow rate brine/RConn1
  Flow Rate Brine Sensor/RConn3 -- Mass flow rate brine/RConn1

== system RM3_Hydraulic_PTO/PTO-Sim - Crankshaft DA 4 Cylinders Try 5 - Cylinder shutoff control - 1/Water Quality Block ==
  A_w/Bs : fl_lib/Physical Signals/Functions/PS Gain  gain=3.812*10^(-12)/(6.986*10^(-8))
  C_m : fl_lib/Physical Signals/Sources/PS Constant  constant=35000
  Constant : Constant  Value=0
  Cp : Scope  NumInputPorts=2
  Divide : Product
  If : If
  If Action Perm Flow  > 0 : Subsystem  TreatAsAtomicUnit=on
  If Action Subsystem1 : Subsystem  TreatAsAtomicUnit=on
  P Permeate Exit : Scope
  PS Add : fl_lib/Physical Signals/Functions/PS Add
  PS Constant : fl_lib/Physical Signals/Sources/PS Constant  constant=1 Pa
  PS Divide : fl_lib/Physical Signals/Functions/PS Divide
      settings: SourceProductName=Simscape  SourceProductBaseCode=SS
  PS Subtract1 : fl_lib/Physical Signals/Functions/PS Subtract
      settings: SourceProductName=Simscape
  PS-Simulink Converter{5..6,8..11} (6 alike) : nesl_utility/PS-Simulink Converter  PhysicalDomain=network_engine_domain  SubClassName=ps_output  LeftPortType=input  RightPortType=output  PseudoPeriodic=off  Frequencies=[]  Unit=inherit  AffineConversion=off
  Permeate Cp*Flow : Scope
  Recov Ratio : fl_lib/Physical Signals/Functions/PS Divide
      settings: SourceProductName=Simscape  SourceProductBaseCode=SS
  Recov Ratio % : Scope
  Pressure Perm Before : PMIOPort  Side=Left
  Pressure Dop Permeate : PMIOPort  Port=2  Side=Left
  Flow rate feed sensor : PMIOPort  Port=3  Side=Left
  Flow rate permeate : PMIOPort  Port=4  Side=Left
  wires:
  If Action Perm Flow  > 0/1(Out1) -> Cp/2
  Divide/1 -> Permeate Cp*Flow/1
  If/1 -> If Action Perm Flow  > 0/Action
  If Action Subsystem1/1(Out1) -> Cp/1
  If/2 -> If Action Subsystem1/Action
  PS-Simulink Converter10/1 -> Divide/1
  PS-Simulink Converter9/1 -> If/1
  PS-Simulink Converter8/1 -> P Permeate Exit/1
  PS-Simulink Converter6/1 -> Recov Ratio %/1
  PS-Simulink Converter11/1 -> Divide/2
  Constant/1 -> If Action Subsystem1/1(In1)
  PS-Simulink Converter5/1 -> If Action Perm Flow  > 0/1(In1)
  connections:
  A_w/Bs/LConn1 -- PS-Simulink Converter9/LConn1 -- PS Subtract1/LConn1 -- Pressure Perm Before/RConn1
  PS Divide/RConn1 -- PS-Simulink Converter5/LConn1 -- PS-Simulink Converter10/LConn1
  Recov Ratio/RConn1 -- PS-Simulink Converter6/LConn1
  PS Constant/RConn1 -- PS Add/LConn2
  Recov Ratio/LConn1 -- PS-Simulink Converter11/LConn1 -- Flow rate permeate/RConn1
  PS Subtract1/RConn1 -- PS-Simulink Converter8/LConn1
  PS Add/LConn1 -- A_w/Bs/RConn1
  C_m/RConn1 -- PS Divide/LConn1
  PS Divide/LConn2 -- PS Add/RConn1
  Flow rate feed sensor/RConn1 -- Recov Ratio/LConn2
  Pressure Dop Permeate/RConn1 -- PS Subtract1/LConn2

== system RM3_Hydraulic_PTO/PTO-Sim - Crankshaft DA Cylinder - doesn't work/Water Quality Block ==
  A_w/Bs : fl_lib/Physical Signals/Functions/PS Gain  gain=3.812*10^(-12)/(6.986*10^(-8))
  C_m : fl_lib/Physical Signals/Sources/PS Constant  constant=35000
  Constant : Constant  Value=0
  Cp : Scope  NumInputPorts=2
  Divide : Product
  If : If
  If Action Perm Flow  > 0 : Subsystem  TreatAsAtomicUnit=on
  If Action Subsystem1 : Subsystem  TreatAsAtomicUnit=on
  P Permeate Exit : Scope
  PS Add : fl_lib/Physical Signals/Functions/PS Add
  PS Constant : fl_lib/Physical Signals/Sources/PS Constant  constant=1 Pa
  PS Divide : fl_lib/Physical Signals/Functions/PS Divide
      settings: SourceProductName=Simscape  SourceProductBaseCode=SS
  PS Subtract1 : fl_lib/Physical Signals/Functions/PS Subtract
      settings: SourceProductName=Simscape
  PS-Simulink Converter{5..6,8..11} (6 alike) : nesl_utility/PS-Simulink Converter  PhysicalDomain=network_engine_domain  SubClassName=ps_output  LeftPortType=input  RightPortType=output  PseudoPeriodic=off  Frequencies=[]  Unit=inherit  AffineConversion=off
  Permeate Cp*Flow : Scope
  Recov Ratio : fl_lib/Physical Signals/Functions/PS Divide
      settings: SourceProductName=Simscape  SourceProductBaseCode=SS
  Recov Ratio % : Scope
  Pressure Perm Before : PMIOPort  Side=Left
  Pressure Dop Permeate : PMIOPort  Port=2  Side=Left
  Flow rate feed sensor : PMIOPort  Port=3  Side=Left
  Flow rate permeate : PMIOPort  Port=4  Side=Left
  wires:
  If Action Perm Flow  > 0/1(Out1) -> Cp/2
  Divide/1 -> Permeate Cp*Flow/1
  If/1 -> If Action Perm Flow  > 0/Action
  If Action Subsystem1/1(Out1) -> Cp/1
  If/2 -> If Action Subsystem1/Action
  PS-Simulink Converter10/1 -> Divide/1
  PS-Simulink Converter9/1 -> If/1
  PS-Simulink Converter8/1 -> P Permeate Exit/1
  PS-Simulink Converter6/1 -> Recov Ratio %/1
  PS-Simulink Converter11/1 -> Divide/2
  Constant/1 -> If Action Subsystem1/1(In1)
  PS-Simulink Converter5/1 -> If Action Perm Flow  > 0/1(In1)
  connections:
  A_w/Bs/LConn1 -- PS-Simulink Converter9/LConn1 -- Pressure Perm Before/RConn1 -- PS Subtract1/LConn1
  PS Divide/RConn1 -- PS-Simulink Converter5/LConn1 -- PS-Simulink Converter10/LConn1
  Recov Ratio/RConn1 -- PS-Simulink Converter6/LConn1
  PS Constant/RConn1 -- PS Add/LConn2
  Recov Ratio/LConn1 -- Flow rate permeate/RConn1 -- PS-Simulink Converter11/LConn1
  PS Subtract1/RConn1 -- PS-Simulink Converter8/LConn1
  PS Add/LConn1 -- A_w/Bs/RConn1
  C_m/RConn1 -- PS Divide/LConn1
  PS Divide/LConn2 -- PS Add/RConn1
  Flow rate feed sensor/RConn1 -- Recov Ratio/LConn2
  Pressure Dop Permeate/RConn1 -- PS Subtract1/LConn2

== system RM3_Hydraulic_PTO/PTO-Sim - Crankshaft DA Cylinder Try 2 - WORKS!1/Hydraulic cylinder and valves ==
  3 Way Directional Valve : sh_lib/Valves/Directional Valves/3-Way Directional Valve  area_spec=sh.valves.directional_valves.enum.area_spec.identical  x_0_P=0 m  x_0_T=0 m  mdl_type_identical=sh.valves.directional_valves.enum.mdl_type.linear  mdl_type_different=sh.valves.directional_valves.enum.mdl_type.linear  opening_max=0.75 in  area_max=pi*(0.75/2)^2 in^2  opening_max_P_A=0.005 m  area_max_P_A=0.5e-4 m^2  opening_max_A_T=0.005 m  area_max_A_T=0.5e-4 m^2  opening_area_tab=[-.002, 0, .002, .005, .015] m  area_tab=[1e-09, 2.0352e-07, 4.0736e-05, .00011438, .00034356] m^2  opening_flow_rate_tab=[-.002, 0, .002, .005, .015] m  pressure_tab=[-10000000, -5000000, -2000000, 2000000, 5000000, 10000000] Pa  flow_rate_tab=[-1e-07, -7.0711e-08, -4.4721e-08, 4.4721e-08, 7.0711e-08, 1e-07; -2.0352e-05, -1.4391e-05, -9.1017e-06, 9.1017e-06, 1.4391e-05, 2.0352e-05; -.0040736, -.0028805, -.0018218, .0018218, .0028805, .0040736; -.011438, -.0080879, -.0051152, .0051152, .0080879, .011438; -.034356, -.024293, -.015364, .015364, .024293, .034356] m^3/s  opening_area_tab_P_A=[-.002, 0, .002, .005, .015] m  area_tab_P_A=[1e-09, 2.0352e-07, 4.0736e-05, .00011438, .00034356] m^2  opening_flow_rate_tab_P_A=[-.002, 0, .002, .005, .015] m  pressure_tab_P_A=[-10000000, -5000000, -2000000, 2000000, 5000000, 10000000] Pa  flow_rate_tab_P_A=[-1e-07, -7.0711e-08, -4.4721e-08, 4.4721e-08, 7.0711e-08, 1e-07; -2.0352e-05, -1.4391e-05, -9.1017e-06, 9.1017e-06, 1.4391e-05, 2.0352e-05; -.0040736, -.0028805, -.0018218, .0018218, .0028805, .0040736; -.011438, -.0080879, -.0051152, .0051152, .0080879, .011438; -.034356, -.024293, -.015364, .015364, .024293, .034356] m^3/s  opening_area_tab_A_T=[-.002, 0, .002, .005, .015] m  area_tab_A_T=[1e-09, 2.0352e-07, 4.0736e-05, .00011438, .00034356] m^2  opening_flow_rate_tab_A_T=[-.002, 0, .002, .005, .015] m  pressure_tab_A_T=[-10000000, -5000000, -2000000, 2000000, 5000000, 10000000] Pa  flow_rate_tab_A_T=[-1e-07, -7.0711e-08, -4.4721e-08, 4.4721e-08, 7.0711e-08, 1e-07; -2.0352e-05, -1.4391e-05, -9.1017e-06, 9.1017e-06, 1.4391e-05, 2.0352e-05; -.0040736, -.0028805, -.0018218, .0018218, .0028805, .0040736; -.011438, -.0080879, -.0051152, .0051152, .0080879, .011438; -.034356, -.024293, -.015364, .015364, .024293, .034356] m^3/s  interp_method_identical=sh.valves.directional_valves.enum.interp_method.linear  interp_method_different=sh.valves.directional_valves.enum.interp_method.linear  extrap_method_identical=sh.valves.directional_valves.enum.extrap_method.linear  extrap_method_different=sh.valves.directional_valves.enum.extrap_method.linear  A_leak=1e-12 m^2  C_d=0.7  lam_spec=sh.valves.directional_valves.enum.lam_spec.pressure_ratio  B_lam=0.999  Re_cr=12
      settings: SourceProductName=Simscape Fluids  SourceProductBaseCode=SH  InternalSimscapePortConfiguration="{\"Bottom\":[],\"Left\":[{\"id\":\"A\",\"label\":\"A\",\"type\":\"foundation.hydraulic.hydraulic\"}],\"Right\":[{\"id\":\"S\",\"label\":\"S\",\"type\":\"input\"},{\"id\":\"P\",\"label\":\"P\",\"type\":\"foundation.hydraulic.hydraulic\"},{\"id\":\"T\",\"label\":\"T\",\"type\":\"foundation.hydraulic.hydraulic\"}],\"Top\":[]}"
  3 Way Directional Valve1 : sh_lib/Valves/Directional Valves/3-Way Directional Valve  area_spec=sh.valves.directional_valves.enum.area_spec.identical  x_0_P=0 m  x_0_T=0 m  mdl_type_identical=sh.valves.directional_valves.enum.mdl_type.linear  mdl_type_different=sh.valves.directional_valves.enum.mdl_type.linear  opening_max=0.75 in  area_max=pi*(0.75/2)^2 in^2  opening_max_P_A=0.005 m  area_max_P_A=0.5e-4 m^2  opening_max_A_T=0.005 m  area_max_A_T=0.5e-4 m^2  opening_area_tab=[-.002, 0, .002, .005, .015] m  area_tab=[1e-09, 2.0352e-07, 4.0736e-05, .00011438, .00034356] m^2  opening_flow_rate_tab=[-.002, 0, .002, .005, .015] m  pressure_tab=[-10000000, -5000000, -2000000, 2000000, 5000000, 10000000] Pa  flow_rate_tab=[-1e-07, -7.0711e-08, -4.4721e-08, 4.4721e-08, 7.0711e-08, 1e-07; -2.0352e-05, -1.4391e-05, -9.1017e-06, 9.1017e-06, 1.4391e-05, 2.0352e-05; -.0040736, -.0028805, -.0018218, .0018218, .0028805, .0040736; -.011438, -.0080879, -.0051152, .0051152, .0080879, .011438; -.034356, -.024293, -.015364, .015364, .024293, .034356] m^3/s  opening_area_tab_P_A=[-.002, 0, .002, .005, .015] m  area_tab_P_A=[1e-09, 2.0352e-07, 4.0736e-05, .00011438, .00034356] m^2  opening_flow_rate_tab_P_A=[-.002, 0, .002, .005, .015] m  pressure_tab_P_A=[-10000000, -5000000, -2000000, 2000000, 5000000, 10000000] Pa  flow_rate_tab_P_A=[-1e-07, -7.0711e-08, -4.4721e-08, 4.4721e-08, 7.0711e-08, 1e-07; -2.0352e-05, -1.4391e-05, -9.1017e-06, 9.1017e-06, 1.4391e-05, 2.0352e-05; -.0040736, -.0028805, -.0018218, .0018218, .0028805, .0040736; -.011438, -.0080879, -.0051152, .0051152, .0080879, .011438; -.034356, -.024293, -.015364, .015364, .024293, .034356] m^3/s  opening_area_tab_A_T=[-.002, 0, .002, .005, .015] m  area_tab_A_T=[1e-09, 2.0352e-07, 4.0736e-05, .00011438, .00034356] m^2  opening_flow_rate_tab_A_T=[-.002, 0, .002, .005, .015] m  pressure_tab_A_T=[-10000000, -5000000, -2000000, 2000000, 5000000, 10000000] Pa  flow_rate_tab_A_T=[-1e-07, -7.0711e-08, -4.4721e-08, 4.4721e-08, 7.0711e-08, 1e-07; -2.0352e-05, -1.4391e-05, -9.1017e-06, 9.1017e-06, 1.4391e-05, 2.0352e-05; -.0040736, -.0028805, -.0018218, .0018218, .0028805, .0040736; -.011438, -.0080879, -.0051152, .0051152, .0080879, .011438; -.034356, -.024293, -.015364, .015364, .024293, .034356] m^3/s  interp_method_identical=sh.valves.directional_valves.enum.interp_method.linear  interp_method_different=sh.valves.directional_valves.enum.interp_method.linear  extrap_method_identical=sh.valves.directional_valves.enum.extrap_method.linear  extrap_method_different=sh.valves.directional_valves.enum.extrap_method.linear  A_leak=1e-12 m^2  C_d=0.7  lam_spec=sh.valves.directional_valves.enum.lam_spec.pressure_ratio  B_lam=0.999  Re_cr=12
      settings: SourceProductName=Simscape Fluids  SourceProductBaseCode=SH  InternalSimscapePortConfiguration="{\"Bottom\":[],\"Left\":[{\"id\":\"A\",\"label\":\"A\",\"type\":\"foundation.hydraulic.hydraulic\"}],\"Right\":[{\"id\":\"S\",\"label\":\"S\",\"type\":\"input\"},{\"id\":\"P\",\"label\":\"P\",\"type\":\"foundation.hydraulic.hydraulic\"},{\"id\":\"T\",\"label\":\"T\",\"type\":\"foundation.hydraulic.hydraulic\"}],\"Top\":[]}"
  Check Valve : sh_lib/Valves/Directional Valves/Check Valve  Commented=on  area_max=pi*(0.75/2)^2 in^2  pres_crack=0.3e5 Pa  pres_max=1.2e5 Pa  C_d=0.7  A_leak=1e-12 m^2  lam_spec=1  B_lam=0.999  Re_cr=12  dynamic=0  tau=0.1 s  area_init=1e-12 m^2
      settings: SourceProductName=Simscape Fluids  SourceProductBaseCode=SH  InternalSimscapePortConfiguration="{\"Bottom\":[],\"Left\":[{\"id\":\"A\",\"label\":\"A\",\"type\":\"foundation.hydraulic.hydraulic\"}],\"Right\":[{\"id\":\"B\",\"label\":\"B\",\"type\":\"foundation.hydraulic.hydraulic\"}],\"Top\":[]}"
  Check Valve1 : sh_lib/Valves/Directional Valves/Check Valve  Commented=on  area_max=pi*(0.75/2)^2 in^2  pres_crack=0.3e5 Pa  pres_max=1.2e5 Pa  C_d=0.7  A_leak=1e-12 m^2  lam_spec=1  B_lam=0.999  Re_cr=12  dynamic=0  tau=0.1 s  area_init=1e-12 m^2
      settings: SourceProductName=Simscape Fluids  SourceProductBaseCode=SH  InternalSimscapePortConfiguration="{\"Bottom\":[],\"Left\":[{\"id\":\"A\",\"label\":\"A\",\"type\":\"foundation.hydraulic.hydraulic\"}],\"Right\":[{\"id\":\"B\",\"label\":\"B\",\"type\":\"foundation.hydraulic.hydraulic\"}],\"Top\":[]}"
  Double-Acting Hydraulic Cylinder (Simple) : sh_lib/Hydraulic Cylinders/Double-Acting Hydraulic Cylinder (Simple)  area_A=0.0025746658 m^2  area_B=0.0025746658 m^2  stroke=12 in  init_pos=5 in  penetr_coeff=1e12 s*N/m^2  or=1
      settings: SourceProductName=Simscape Fluids  SourceProductBaseCode=SH  InternalSimscapePortConfiguration="{\"Bottom\":[],\"Left\":[{\"id\":\"C\",\"label\":\"C\",\"type\":\"foundation.mechanical.translational.translational\"},{\"id\":\"A\",\"label\":\"A\",\"type\":\"foundation.hydraulic.hydraulic\"}],\"Right\":[{\"id\":\"R\",\"label\":\"R\",\"type\":\"foundation.mechanical.translational.translational\"},{\"id\":\"B\",\"label\":\"B\",\"type\":\"foundation.hydraulic.hydraulic\"}],\"Top\":[]}"
  Ideal Force Sensor : fl_lib/Mechanical/Mechanical Sensors/Ideal Force Sensor
  Ideal Translational Velocity Source : fl_lib/Mechanical/Mechanical Sources/Ideal Translational Velocity Source
  Mechanical Translational Reference : fl_lib/Mechanical/Translational Elements/Mechanical Translational Reference
  Mechanical Translational Reference1 : fl_lib/Mechanical/Translational Elements/Mechanical Translational Reference
  PS Gain : fl_lib/Physical Signals/Functions/PS Gain  gain=-1
  PS-Simulink Converter : nesl_utility/PS-Simulink Converter  PhysicalDomain=network_engine_domain  SubClassName=ps_output  LeftPortType=input  RightPortType=output  PseudoPeriodic=off  Frequencies=[]  Unit=N  AffineConversion=off
  PS-Simulink Converter2 : nesl_utility/PS-Simulink Converter  PhysicalDomain=network_engine_domain  SubClassName=ps_output  LeftPortType=input  RightPortType=output  PseudoPeriodic=off  Frequencies=[]  Unit=inherit  AffineConversion=off
  Relay : Relay  OnSwitchValue=0  OffSwitchValue=0  OffOutputValue=-1
  Simulink-PS Converter1 : nesl_utility/Simulink-PS Converter  PhysicalDomain=network_engine_domain  SubClassName=ps_input  LeftPortType=input  RightPortType=output  PseudoPeriodic=off  Frequencies=[]  NoiseDistribution=none  NoiseParameters=[]  Unit=1  AffineConversion=off  FilteringAndDerivatives=zero  SimscapeFilterOrder=1  InputFilterTimeConstant=0.001  UdotUserProvided=0
  Velocity input : PMIOPort  Side=Left
  Flow out : PMIOPort  Port=2  Side=Left
  Seawater In : PMIOPort  Port=3  Side=Left
  Force Out : Outport
  wires:
  PS-Simulink Converter2/1 -> Relay/1
  Relay/1 -> Simulink-PS Converter1/1
  PS-Simulink Converter/1 -> Force Out/1
  connections:
  Ideal Translational Velocity Source/LConn1 -- Double-Acting Hydraulic Cylinder (Simple)/RConn1
  3 Way Directional Valve1/RConn2 -- 3 Way Directional Valve/RConn2 -- Seawater In/RConn1
  3 Way Directional Valve/RConn3 -- 3 Way Directional Valve1/RConn3 -- Flow out/RConn1
  3 Way Directional Valve/LConn1 -- Double-Acting Hydraulic Cylinder (Simple)/LConn2
  Simulink-PS Converter1/RConn1 -- PS Gain/LConn1 -- 3 Way Directional Valve/RConn1
  Ideal Translational Velocity Source/RConn1 -- PS-Simulink Converter2/LConn1 -- Velocity input/RConn1
  Ideal Translational Velocity Source/RConn2 -- Mechanical Translational Reference1/LConn1
  Double-Acting Hydraulic Cylinder (Simple)/RConn2 -- 3 Way Directional Valve1/LConn1
  PS Gain/RConn1 -- 3 Way Directional Valve1/RConn1
  Ideal Force Sensor/RConn2 -- PS-Simulink Converter/LConn1
  Ideal Force Sensor/RConn1 -- Mechanical Translational Reference/LConn1
  Ideal Force Sensor/LConn1 -- Double-Acting Hydraulic Cylinder (Simple)/LConn1
